simulink model "Actuator"  (R2024a)
settings: Solver=FixedStepDiscrete  StartTime=0.0  StopTime=10.0  RelTol=1e-3  EnableMultiTasking=on
settings Model: DataDictionary=dict.sldd  Creator=Administrator  LastModifiedBy=Administrator
settings OptimizationCC: DefaultParameterBehavior=Inlined  EnhancedBackFolding=on  PassReuseOutputArgsAs=Individual arguments  ZeroExternalMemoryAtStartup=off  ZeroInternalMemoryAtStartup=off  OptimizeBlockOrder=speed  DifferentSizesBufferReuse=on  OptimizationCustomize=off  EfficientTunableParamExpr=on
settings DebuggingCC: ParameterTunabilityLossMsg=error
settings SFSimCC: MATLABDynamicMemAlloc=off
settings RTWCC: Description=AUTOSAR  SystemTargetFile=autosar.tlc  GenCodeOnly=on  TemplateMakefile=ert_default_tmf  DataTypeReplacement=CDataTypesFixedWidth
settings CodeAppCC: ForceParamTrailComments=on  IgnoreCustomStorageClasses=off  OperatorAnnotations=on  SimulinkDataObjDesc=on  SFDataObjDesc=on  InsertBlockDesc=on
settings STFCustomTargetCC: MultiwordLength=256  ParMdlRefBuildCompliant=on  CompOptLevelCompliant=on  IncludeMdlTerminateFcn=off  CombineOutputUpdateFcns=on  SuppressErrorStatus=on  ERTCustomFileBanners=on  SupportNonFinite=off  SupportComplex=off  SupportContinuousTime=off  SupportNonInlinedSFcns=off  RemoveResetFunc=on  MATLABClassNameForMDSCustomization=Simulink.SoftwareTarget.ERTCustomization  AutosarCompliant=on  GRTInterface=off  LookupTableObjectStructAxisOrder=2,1,3,4,...  LUTObjectStructOrderEvenSpacing=Size,Table,Breakpoints  SystemTargetFile=autosar.tlc
settings ERTTargetCC: TargetLangStandard=C99 (ISO)  ConcurrentExecutionCompliant=off  IncludeMdlTerminateFcn=off  SuppressErrorStatus=on  SupportNonFinite=off  SupportComplex=off  ModelStepFunctionPrototypeControlCompliant=off  CPPClassGenCompliant=off  AutosarCompliant=on  LookupTableObjectStructAxisOrder=2,1,3,4,...  LUTObjectStructOrderEvenSpacing=Size,Table,Breakpoints  InlinedParameterPlacement=NonHierarchical  ERTCustomFileTemplate=example_file_process.tlc  BooleanTrueId=TRUE  BooleanFalseId=FALSE

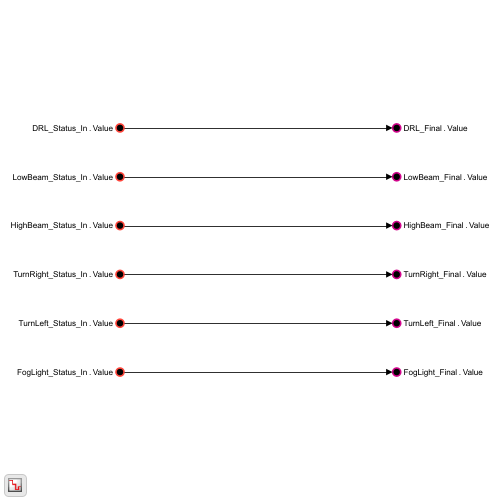
[thumbnail: Simulink's stored preview of the top-level diagram]
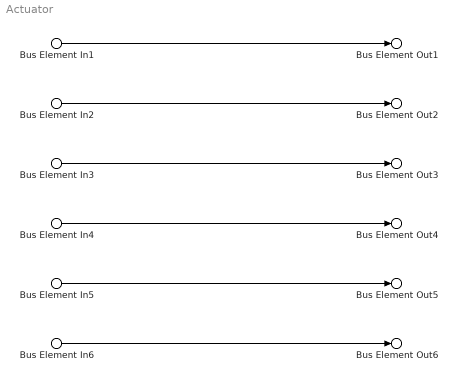
== system Actuator ==
  Bus Element In1 : Inport  Description=|  PortName=DRL_Status_In  Element=Value
      | Lights state On or OFF (LowBeam, HighBeam, DRL, FogLight, ...):
      | 0: Light should be OFF
      | 1: Light should be ON
  Bus Element In2 : Inport  Description=|  Port=2  PortName=LowBeam_Status_In  Element=Value
      | Lights state On or OFF (LowBeam, HighBeam, DRL, FogLight, ...):
      | 0: Light should be OFF
      | 1: Light should be ON
  Bus Element In3 : Inport  Description=|  Port=3  PortName=HighBeam_Status_In  Element=Value
      | Lights state On or OFF (LowBeam, HighBeam, DRL, FogLight, ...):
      | 0: Light should be OFF
      | 1: Light should be ON
  Bus Element In4 : Inport  Description=|  Port=4  PortName=TurnRight_Status_In  Element=Value
      | Lights state On or OFF (LowBeam, HighBeam, DRL, FogLight, ...):
      | 0: Light should be OFF
      | 1: Light should be ON
  Bus Element In5 : Inport  Description=|  Port=5  PortName=TurnLeft_Status_In  Element=Value
      | Lights state On or OFF (LowBeam, HighBeam, DRL, FogLight, ...):
      | 0: Light should be OFF
      | 1: Light should be ON
  Bus Element In6 : Inport  Description=|  Port=6  PortName=FogLight_Status_In  Element=Value
      | Lights state On or OFF (LowBeam, HighBeam, DRL, FogLight, ...):
      | 0: Light should be OFF
      | 1: Light should be ON
  Bus Element Out1 : Outport  PortName=DRL_Final  Element=Value
  Bus Element Out2 : Outport  Port=2  PortName=LowBeam_Final  Element=Value
  Bus Element Out3 : Outport  Port=3  PortName=HighBeam_Final  Element=Value
  Bus Element Out4 : Outport  Port=4  PortName=TurnRight_Final  Element=Value
  Bus Element Out5 : Outport  Port=5  PortName=TurnLeft_Final  Element=Value
  Bus Element Out6 : Outport  Port=6  PortName=FogLight_Final  Element=Value
  wires:
  Bus Element In1/1 -> Bus Element Out1/1
  Bus Element In2/1 -> Bus Element Out2/1
  Bus Element In3/1 -> Bus Element Out3/1
  Bus Element In4/1 -> Bus Element Out4/1
  Bus Element In5/1 -> Bus Element Out5/1
  Bus Element In6/1 -> Bus Element Out6/1
